simulink model "biped_sim_interactive"  (R2016b)
settings: Solver=FixedStepAuto  StartTime=0.0  StopTime=inf  FixedStep=Ts_dynamics  MaxStep=Ts  MinStep=Ts/4  RelTol=1e-3  EnableMultiTasking=on
PreLoadFcn:
  | clear
  | biped_setup
values from neighbouring files (symbols this model uses):
  cstate0 = ControllerState()    [biped_setup.m]
  env = struct()    [BipedController.m]    (also in biped_setup.m = Environment())
  robot = RobotParams()    [Planner.m]
  Ts = 1e-3    (= 0.001)    [BipedController.m]    (also in Planner.m = 0.1; Sequencing.m; StateEstimator.m)
  Ts_controller = 1e-3    (= 0.001)    [biped_setup.m]
  Ts_planner = 1e-1    (= 0.1)    [biped_setup.m]
  X0 = struct()    [RobotState.m]    (also in biped_setup.m = RobotState())
undefined symbols (not defined in the file or in its folder): Control, ControllerParams, RobotParams, RobotState
settings Model: Creator=patrick  LastModifiedBy=robot
settings SolverCC: InitialStep=Ts  InsertRTBMode=Always
settings DataIOCC: SaveOutput=off  SaveTime=off
settings OptimizationCC: LifeSpan=inf
settings DebuggingCC: ReadBeforeWriteMsg=DisableAll  WriteAfterWriteMsg=DisableAll  WriteAfterReadMsg=DisableAll  MultiTaskDSMMsg=none  UnnecessaryDatatypeConvMsg=warning  VectorMatrixConversionMsg=warning  BusObjectLabelMismatch=none  AllowSymbolicDim=off  SFUnexpectedBacktrackingDiag=warning  SFNoUnconditionalDefaultTransitionDiag=warning  SFExecutionAtInitializationDiag=none
settings ModelReferenceCC: UpdateModelReferenceTargets=IfOutOfDate  PropagateSignalLabelsOutOfModel=off
settings SFSimCC: SFSimEcho=off
settings RTWCC: BuildConfiguration=Faster Runs
settings GRTTargetCC: TargetLangStandard=C89/C90 (ANSI)
settings ConfigComp: CovMetricSettings=dw  CovHtmlReporting=on  CovSaveCumulativeToWorkspaceVar=on  CovSaveSingleToWorkspaceVar=on  CovExternalEMLEnable=off

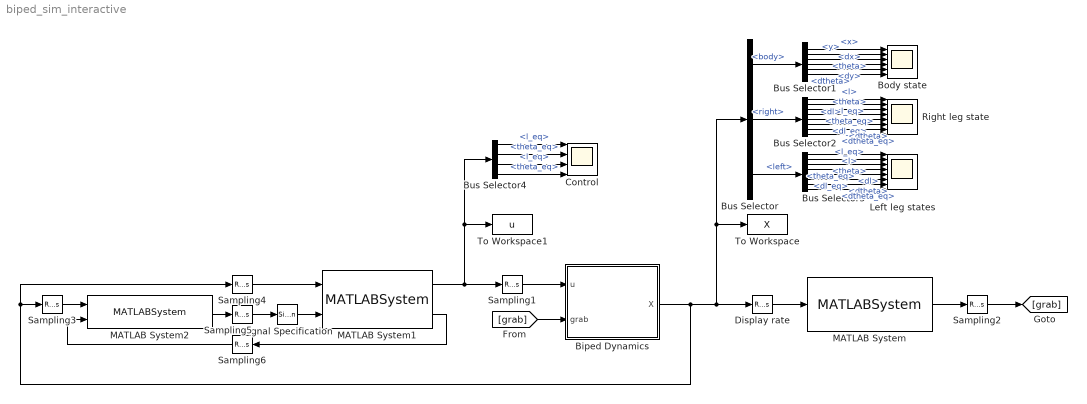
== system biped_sim_interactive ==
  Biped Dynamics : Subsystem
  Body state : Scope  NumInputPorts=6
  Bus Selector : BusSelector  OutputSignals=body,right,left
  Bus Selector1 : BusSelector  OutputSignals=x,y,theta,dx,dy,dtheta
  Bus Selector2 : BusSelector  OutputSignals=l,l_eq,theta,theta_eq,dl,dl_eq,dtheta,dtheta_eq
  Bus Selector3 : BusSelector  OutputSignals=l,l_eq,theta,theta_eq,dl,dl_eq,dtheta,dtheta_eq
  Bus Selector4 : BusSelector  OutputSignals=right.l_eq,right.theta_eq,left.l_eq,left.theta_eq
  Control : Scope  NumInputPorts=4
  Display rate : RateTransition  X0=RobotState()  OutPortSampleTime=Ts_visualization
  Left leg states : Scope  NumInputPorts=8
  MATLAB System : MATLABSystem  System=BipedVisualization  ground_data=env.ground_data  SimulateUsing=Interpreted execution
      mask Type: BipedVisualization
      mask Display:
      | disp('BipedVisualization');
      | port_label('input',1,'X');
      | port_label('output',1,'v');
  MATLAB System1 : MATLABSystem  System=BipedController  Ts=Ts_controller  SimulateUsing=Code generation
      mask Type: BipedController
      mask Display:
      | disp('BipedController');
      | port_label('input',1,'X');
      | port_label('input',2,'cparams');
      | port_label('output',1,'u');
      | port_label('output',2,'cstate');
  MATLAB System2 : MATLABSystem  System=Planner  Ts=Ts_planner  Ts_sim=Ts_sim  robot=RobotParams()  ground_data=env.ground_data  rollout_depth=2  target_dx=1  energy_injection=0  phase_rate=1.5  max_stride=0.4  step_height=0.1  phase_stretch=0  SimulateUsing=Interpreted execution
      mask Type: Planner
      mask Display:
      | disp('Planner');
      | port_label('input',1,'X');
      | port_label('input',2,'cstate');
      | port_label('output',1,'cparams');
  Right leg state : Scope  NumInputPorts=8
  Sampling1 : RateTransition  X0=Control()  OutPortSampleTimeOpt=Inherit  OutPortSampleTime=-2
  Sampling2 : RateTransition  OutPortSampleTimeOpt=Inherit  OutPortSampleTime=Ts/16
  Sampling3 : RateTransition  X0=X0  OutPortSampleTime=Ts_planner
  Sampling4 : RateTransition  X0=X0  OutPortSampleTimeOpt=Inherit  OutPortSampleTime=Ts
  Sampling5 : RateTransition  X0=ControllerParams()  OutPortSampleTime=Ts_controller
  Sampling6 : RateTransition  X0=cstate0  OutPortSampleTimeOpt=Inherit  OutPortSampleTime=Ts
  Signal Specification : SignalSpecification  OutDataTypeStr=Bus: controller_params_bus  Dimensions=[1 1]  BusOutputAsStruct=on
  To Workspace : ToWorkspace  VariableName=X  SaveFormat=Timeseries  SampleTime=-1
      settings: MaxDataPoints=1e6
  To Workspace1 : ToWorkspace  VariableName=u  SaveFormat=Timeseries  SampleTime=-1
      settings: MaxDataPoints=1e6
  wires:
  MATLAB System1/1 -> Sampling1/1, Bus Selector4/1, To Workspace1/1
  Biped Dynamics/1(X) -> Sampling4/1, Sampling3/1, Bus Selector/1, To Workspace/1, Display rate/1
  [grab] -> Biped Dynamics/2(grab)
  MATLAB System/1 -> Sampling2/1
  Display rate/1 -> MATLAB System/1
  Bus Selector/1 -> Bus Selector1/1  "<body>"
  Bus Selector1/1 -> Body state/1  "<x>"
  Bus Selector1/2 -> Body state/2  "<y>"
  Bus Selector1/3 -> Body state/3  "<theta>"
  Bus Selector1/4 -> Body state/4  "<dx>"
  Bus Selector1/5 -> Body state/5  "<dy>"
  Bus Selector1/6 -> Body state/6  "<dtheta>"
  Bus Selector/2 -> Bus Selector2/1  "<right>"
  Bus Selector2/1 -> Right leg state/1  "<l>"
  Bus Selector2/2 -> Right leg state/2  "<l_eq>"
  Bus Selector2/3 -> Right leg state/3  "<theta>"
  Bus Selector2/4 -> Right leg state/4  "<theta_eq>"
  Bus Selector2/5 -> Right leg state/5  "<dl>"
  Bus Selector2/6 -> Right leg state/6  "<dl_eq>"
  Bus Selector2/7 -> Right leg state/7  "<dtheta>"
  Bus Selector2/8 -> Right leg state/8  "<dtheta_eq>"
  Bus Selector/3 -> Bus Selector3/1  "<left>"
  Bus Selector3/1 -> Left leg states/1  "<l>"
  Bus Selector3/2 -> Left leg states/2  "<l_eq>"
  Bus Selector3/3 -> Left leg states/3  "<theta>"
  Bus Selector3/4 -> Left leg states/4  "<theta_eq>"
  Bus Selector3/5 -> Left leg states/5  "<dl>"
  Bus Selector3/6 -> Left leg states/6  "<dl_eq>"
  Bus Selector3/7 -> Left leg states/7  "<dtheta>"
  Bus Selector3/8 -> Left leg states/8  "<dtheta_eq>"
  Sampling2/1 -> [grab]
  Sampling1/1 -> Biped Dynamics/1(u)
  Sampling3/1 -> MATLAB System2/1
  Sampling4/1 -> MATLAB System1/1
  MATLAB System2/1 -> Sampling5/1
  MATLAB System1/2 -> Sampling6/1
  Sampling5/1 -> Signal Specification/1
  Sampling6/1 -> MATLAB System2/2
  Signal Specification/1 -> MATLAB System1/2
  Bus Selector4/1 -> Control/1  "<l_eq>"
  Bus Selector4/2 -> Control/2  "<theta_eq>"
  Bus Selector4/3 -> Control/3  "<l_eq>"
  Bus Selector4/4 -> Control/4  "<theta_eq>"

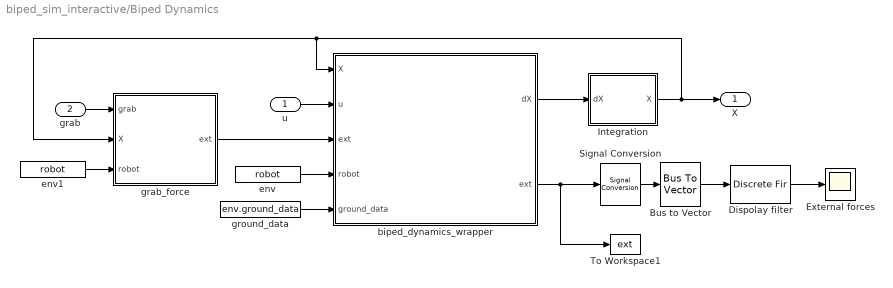
== system biped_sim_interactive/Biped Dynamics ==
  u : Inport
  grab : Inport  Port=2
  Bus to Vector : BusToVector
  Dispolay filter : DiscreteFir
  External forces : Scope
  Integration : Subsystem
  Signal Conversion : SignalConversion  ConversionOutput=Virtual bus  OverrideOpt=off
  To Workspace1 : ToWorkspace  VariableName=ext  SaveFormat=Timeseries  SampleTime=-1
      settings: MaxDataPoints=1e6
  biped_dynamics_wrapper : MATLAB Function  TreatAsAtomicUnit=on
  env : Constant  Value=robot  OutDataTypeStr=Bus: robot_params_bus
  env1 : Constant  Value=robot  OutDataTypeStr=Bus: robot_params_bus
  grab_force : MATLAB Function  TreatAsAtomicUnit=on
  ground_data : Constant  Value=env.ground_data
  X : Outport
  wires:
  u/1 -> biped_dynamics_wrapper/2(u)
  env/1 -> biped_dynamics_wrapper/4(robot)
  ground_data/1 -> biped_dynamics_wrapper/5(ground_data)
  grab/1 -> grab_force/1(grab)
  grab_force/1(ext) -> biped_dynamics_wrapper/3("ext ")
  env1/1 -> grab_force/3(robot)
  Integration/1(X) -> X/1, grab_force/2(X), biped_dynamics_wrapper/1(X)
  biped_dynamics_wrapper/1(dX) -> Integration/1(dX)
  Signal Conversion/1 -> Bus to Vector/1
  biped_dynamics_wrapper/2(ext) -> To Workspace1/1, Signal Conversion/1
  Bus to Vector/1 -> Dispolay filter/1
  Dispolay filter/1 -> External forces/1

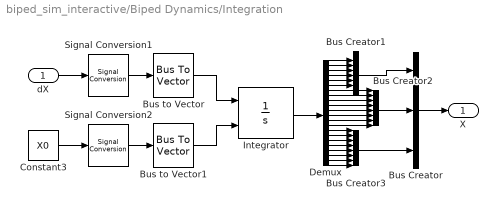
== system biped_sim_interactive/Biped Dynamics/Integration ==
  dX : Inport
  Bus Creator : BusCreator  Inputs=3  OutDataTypeStr=Bus: robot_state_bus  NonVirtualBus=on
      settings: InheritFromInputs=off
  Bus Creator1 : BusCreator  Inputs=6  OutDataTypeStr=Bus: body_state_bus  NonVirtualBus=on
      settings: InheritFromInputs=off
  Bus Creator2 : BusCreator  Inputs=8  OutDataTypeStr=Bus: leg_state_bus  NonVirtualBus=on
      settings: InheritFromInputs=off
  Bus Creator3 : BusCreator  Inputs=8  OutDataTypeStr=Bus: leg_state_bus  NonVirtualBus=on
      settings: InheritFromInputs=off
  Bus to Vector : BusToVector
  Bus to Vector1 : BusToVector
  Constant3 : Constant  Value=X0  OutDataTypeStr=Bus: robot_state_bus
  Demux : Demux  Outputs=22
  Integrator : Integrator  InitialConditionSource=external  InitialCondition=X0
  Signal Conversion1 : SignalConversion  ConversionOutput=Virtual bus  OverrideOpt=off
  Signal Conversion2 : SignalConversion  ConversionOutput=Virtual bus  OverrideOpt=off
  X : Outport
  wires:
  Bus to Vector/1 -> Integrator/1
  Bus to Vector1/1 -> Integrator/2
  Constant3/1 -> Signal Conversion2/1
  Signal Conversion1/1 -> Bus to Vector/1
  Signal Conversion2/1 -> Bus to Vector1/1
  dX/1 -> Signal Conversion1/1
  Integrator/1 -> Demux/1
  Bus Creator/1 -> X/1
  Demux/1 -> Bus Creator1/1
  Demux/2 -> Bus Creator1/2
  Demux/3 -> Bus Creator1/3
  Demux/4 -> Bus Creator1/4
  Demux/5 -> Bus Creator1/5
  Demux/6 -> Bus Creator1/6
  Demux/7 -> Bus Creator2/1
  Demux/8 -> Bus Creator2/2
  Demux/9 -> Bus Creator2/3
  Demux/10 -> Bus Creator2/4
  Demux/11 -> Bus Creator2/5
  Demux/12 -> Bus Creator2/6
  Demux/13 -> Bus Creator2/7
  Demux/14 -> Bus Creator2/8
  Demux/15 -> Bus Creator3/1
  Demux/16 -> Bus Creator3/2
  Demux/17 -> Bus Creator3/3
  Demux/18 -> Bus Creator3/4
  Demux/19 -> Bus Creator3/5
  Demux/20 -> Bus Creator3/6
  Demux/21 -> Bus Creator3/7
  Demux/22 -> Bus Creator3/8
  Bus Creator3/1 -> Bus Creator/3
  Bus Creator2/1 -> Bus Creator/2
  Bus Creator1/1 -> Bus Creator/1

== matlab function biped_sim_interactive/Biped Dynamics/biped_dynamics_wrapper ==
  data: X input Bus: robot_state_bus; u input Bus: control_bus; dX output Bus: robot_state_bus; ext input Bus: external_force_bus; robot input Bus: robot_params_bus; ground_data input; ext output
function [dX, ext] = biped_dynamics_wrapper(X, u, ext, robot, ground_data) %#codegen

% Get local terrain
env = Environment(ground_data);
terrain = env.getLocalTerrain(X.body.x);

% Compute derivatives
[dX, ext] = biped_dynamics(X, u, ext, robot, terrain);

== matlab function biped_sim_interactive/Biped Dynamics/grab_force ==
  data: grab input; ext output Bus: external_force_bus; X input Bus: robot_state_bus; robot input Bus: robot_params_bus
function ext = grab_force(grab, X, robot) %#codegen

kp_f_ext = 1e4;
kd_f_ext = 2*sqrt(kp_f_ext*robot.body.mass);
 
ext.body.x     = 0;
ext.body.y     = 0;
ext.body.theta = 0;
ext.right.x    = 0;
ext.right.y    = 0;
ext.left.x     = 0;
ext.left.y     = 0;

if any(grab ~= 0)
    ext.body.x = (kp_f_ext * grab(1)) - (kd_f_ext * X.body.dx);
    ext.body.y = (kp_f_ext * grab(2)) - (kd_f_ext * X.body.dy);
end
